simulink model "obserwator_stanu"  (R2022b)
settings: Solver=ode3  StartTime=0.0  StopTime=1  FixedStep=Tp  RelTol=1e-3
values from neighbouring files (symbols this model uses):
  A = [0 1 0; a21 0 a23; a31 0 a33]    [init.m]    (also in proj.m)
  a21 = 1/2/m * x30^2 * FemP1/FemP2^2 * exp(-x10/FemP2)    [init.m]    (also in proj.m)
  a23 = -1/m * x30 * FemP1/FemP2 * exp(-x10/FemP2)    [init.m]    (also in proj.m)
  a31 = 1/f1 * exp(x10/f2) * (ki*u10 + ci - x30)    [init.m]    (also in proj.m)
  a33 = -f2/f1 * exp(x10/f2)    [init.m]    (also in proj.m)
  B = [0 0; 0 g; b31 0]    [init.m]    (also in proj.m)
  b31 = ki * f2/f1 * exp(x10/f2)    [init.m]    (also in proj.m)
  C = [1 0 0]    [init.m]    (also in proj.m)
  g = 9.81    [init.m]    (also in proj.m)
  K = place(A, B(:, 1), [-28, -60, -90])    [init.m]    (also in proj.m)
  L = acker(A', C', p)'    [init.m]    (also in proj.m)
  Tp = 0.00001    (= 1e-05)    [init.m]    (also in proj.m)
  xd = d-bd    [init.m]    (also in proj.m)
settings Model: Creator=TheZl  LastModifiedBy=minekuba

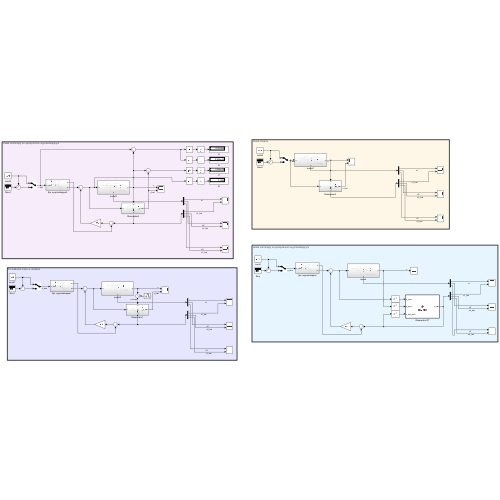
[thumbnail: Simulink's stored preview of the top-level diagram]
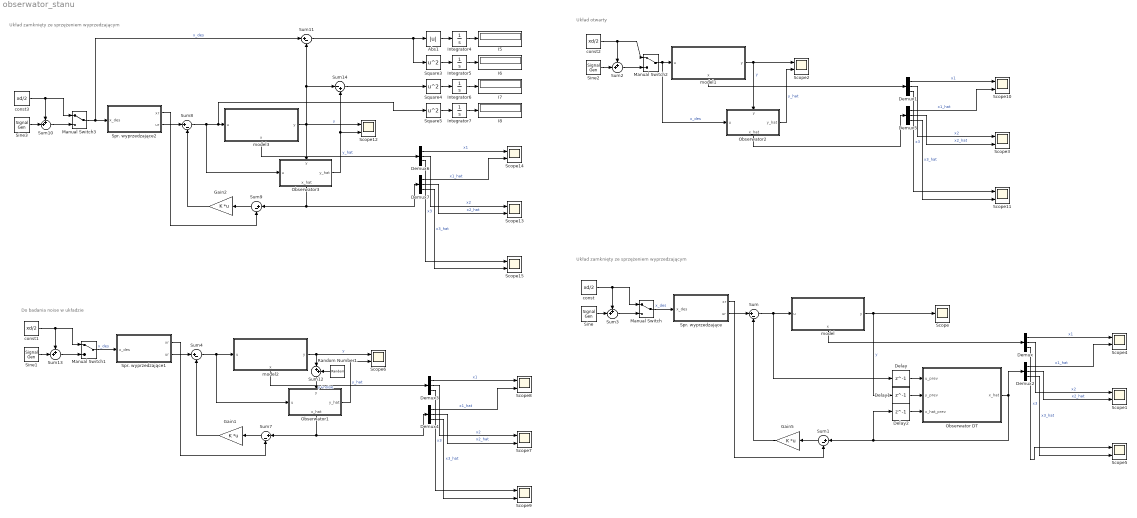
== system obserwator_stanu ==
  note: Układ zamknięty ze sprzężeniem wyprzedzającym
  note: Do badania noise w układzie
  note: Układ otwarty
  note: Układ zamknięty ze sprzężeniem wyprzedzającym
  Abs1 : Abs  SaturateOnIntegerOverflow=off
  Delay : Delay  DelayLength=1
  Delay1 : Delay  DelayLength=1
  Delay2 : Delay  DelayLength=1  InitialCondition=[0 0 0]'
  Demux{,1..7} (8 alike) : Demux  Outputs=3
  Gain1 : Gain  Gain=K  Multiplication=Matrix(K*u)
  Gain2 : Gain  Gain=K  Multiplication=Matrix(K*u)
  Gain5 : Gain  Gain=K  Multiplication=Matrix(K*u)
  I{5..8} (4 alike) : Display
  Integrator{4..7} (4 alike) : Integrator
  Manual Switch{,1..3} (4 alike) : ManualSwitch
  Obserwator DT : MATLAB Function  TreatAsAtomicUnit=on
  Obserwator1 : Subsystem
      settings: PortSchema="{\"entries\":[{\"content\":{\"sides\":[{\"content\":{\"connectorIds\":[\"In1\"]},\"type\":\"ConnectorPlacement.EquallySpacedRectSide\",\"uuid\":\"f0864749-42ee-43af-89d8-e79f181d54f0\"},{\"content\":{\"connectorIds\":[\"Out1\"],\"side\":\"RIGHT\"},\"type\":\"ConnectorPlacement.EquallySpacedRectSide\",\"uuid\":\"0332ef02-e2af-4e04-af5b-f19b3f506f90\"},{\"content\":{\"connectorIds\":[\"In2\"],\"side\":\"TOP\"},\"type\":\"ConnectorPlacement.EquallySpacedRectSide\",\"uuid\":\"17939e36-b316-45a4-8ef0-4ca25066d29d\"},{\"content\":{\"connectorIds\":[\"Out2\"],\"side\":\"BOTTOM\"},\"type\":\"ConnectorPlacement.EquallySpacedRectSide\",\"uuid\":\"291cc938-6a40-4d14-9d0d-6f037a5c762b\"}]},\"type\":\"ConnectorPlacement.EquallySpacedConnector\",\"uuid\":\"9ac518b4-bfcb-4f10-b20b-cf60c9eac4c7\"}],\"packageUris\":[\"http://schema.mathworks.com/mf0/Connector/R2020b\"],\"version\":\"1.0\"}"
  Obserwator2 : Subsystem
      settings: PortSchema="{\"entries\":[{\"content\":{\"sides\":[{\"content\":{\"connectorIds\":[\"In1\"]},\"type\":\"ConnectorPlacement.EquallySpacedRectSide\",\"uuid\":\"f0864749-42ee-43af-89d8-e79f181d54f0\"},{\"content\":{\"connectorIds\":[\"Out1\"],\"side\":\"RIGHT\"},\"type\":\"ConnectorPlacement.EquallySpacedRectSide\",\"uuid\":\"0332ef02-e2af-4e04-af5b-f19b3f506f90\"},{\"content\":{\"connectorIds\":[\"In2\"],\"side\":\"TOP\"},\"type\":\"ConnectorPlacement.EquallySpacedRectSide\",\"uuid\":\"17939e36-b316-45a4-8ef0-4ca25066d29d\"},{\"content\":{\"connectorIds\":[\"Out2\"],\"side\":\"BOTTOM\"},\"type\":\"ConnectorPlacement.EquallySpacedRectSide\",\"uuid\":\"291cc938-6a40-4d14-9d0d-6f037a5c762b\"}]},\"type\":\"ConnectorPlacement.EquallySpacedConnector\",\"uuid\":\"9ac518b4-bfcb-4f10-b20b-cf60c9eac4c7\"}],\"packageUris\":[\"http://schema.mathworks.com/mf0/Connector/R2020b\"],\"version\":\"1.0\"}"
  Obserwator3 : Subsystem
      settings: PortSchema="{\"entries\":[{\"content\":{\"sides\":[{\"content\":{\"connectorIds\":[\"In1\"]},\"type\":\"ConnectorPlacement.EquallySpacedRectSide\",\"uuid\":\"f0864749-42ee-43af-89d8-e79f181d54f0\"},{\"content\":{\"connectorIds\":[\"Out1\"],\"side\":\"RIGHT\"},\"type\":\"ConnectorPlacement.EquallySpacedRectSide\",\"uuid\":\"0332ef02-e2af-4e04-af5b-f19b3f506f90\"},{\"content\":{\"connectorIds\":[\"In2\"],\"side\":\"TOP\"},\"type\":\"ConnectorPlacement.EquallySpacedRectSide\",\"uuid\":\"17939e36-b316-45a4-8ef0-4ca25066d29d\"},{\"content\":{\"connectorIds\":[\"Out2\"],\"side\":\"BOTTOM\"},\"type\":\"ConnectorPlacement.EquallySpacedRectSide\",\"uuid\":\"291cc938-6a40-4d14-9d0d-6f037a5c762b\"}]},\"type\":\"ConnectorPlacement.EquallySpacedConnector\",\"uuid\":\"9ac518b4-bfcb-4f10-b20b-cf60c9eac4c7\"}],\"packageUris\":[\"http://schema.mathworks.com/mf0/Connector/R2020b\"],\"version\":\"1.0\"}"
  Random Number1 : RandomNumber  Variance=1e-5
  Scope : Scope
  Scope{1..15} (15 alike) : Scope  NumInputPorts=2
  Sine{,1..3} (4 alike) : SignalGenerator  Amplitude=xd/12  Frequency=0.2
  Spr. wyprzedzające : Subsystem
  Spr. wyprzedzające1 : Subsystem
  Spr. wyprzedzające2 : Subsystem
  Square3 : Math  Operator=square
  Square4 : Math  Operator=square
  Square5 : Math  Operator=square
  Sum{,1,4,7..9,11} (7 alike) : Sum  Inputs=|+-
  Sum{2..3,10,13} (4 alike) : Sum  Inputs=++|
  Sum12 : Sum  Inputs=|++
  Sum14 : Sum  Inputs=|-+
  const{,1..3} (4 alike) : Constant  Value=xd/2
  model : Subsystem
      settings: PortSchema="{\"entries\":[{\"content\":{\"sides\":[{\"content\":{\"connectorIds\":[\"In1\"]},\"type\":\"ConnectorPlacement.EquallySpacedRectSide\",\"uuid\":\"08100310-f669-4bec-b75a-4c341ab1329c\"},{\"content\":{\"connectorIds\":[\"Out1\"],\"side\":\"RIGHT\"},\"type\":\"ConnectorPlacement.EquallySpacedRectSide\",\"uuid\":\"75a75395-bc88-4968-acfb-02365cdbbaac\"},{\"content\":{\"connectorIds\":[],\"side\":\"TOP\"},\"type\":\"ConnectorPlacement.EquallySpacedRectSide\",\"uuid\":\"7e90434d-1931-47ff-b270-f1d54f71bb7e\"},{\"content\":{\"connectorIds\":[\"Out2\"],\"side\":\"BOTTOM\"},\"type\":\"ConnectorPlacement.EquallySpacedRectSide\",\"uuid\":\"09ce4af7-043c-4542-961c-50c1fb378fc1\"}]},\"type\":\"ConnectorPlacement.EquallySpacedConnector\",\"uuid\":\"9c93e3e1-5fb5-4a02-9a28-f46059e1f065\"}],\"packageUris\":[\"http://schema.mathworks.com/mf0/Connector/R2020b\"],\"version\":\"1.0\"}"
  model1 : Subsystem
      settings: PortSchema="{\"entries\":[{\"content\":{\"sides\":[{\"content\":{\"connectorIds\":[\"In1\"]},\"type\":\"ConnectorPlacement.EquallySpacedRectSide\",\"uuid\":\"08100310-f669-4bec-b75a-4c341ab1329c\"},{\"content\":{\"connectorIds\":[\"Out1\"],\"side\":\"RIGHT\"},\"type\":\"ConnectorPlacement.EquallySpacedRectSide\",\"uuid\":\"75a75395-bc88-4968-acfb-02365cdbbaac\"},{\"content\":{\"connectorIds\":[],\"side\":\"TOP\"},\"type\":\"ConnectorPlacement.EquallySpacedRectSide\",\"uuid\":\"7e90434d-1931-47ff-b270-f1d54f71bb7e\"},{\"content\":{\"connectorIds\":[\"Out2\"],\"side\":\"BOTTOM\"},\"type\":\"ConnectorPlacement.EquallySpacedRectSide\",\"uuid\":\"09ce4af7-043c-4542-961c-50c1fb378fc1\"}]},\"type\":\"ConnectorPlacement.EquallySpacedConnector\",\"uuid\":\"9c93e3e1-5fb5-4a02-9a28-f46059e1f065\"}],\"packageUris\":[\"http://schema.mathworks.com/mf0/Connector/R2020b\"],\"version\":\"1.0\"}"
  model2 : Subsystem
      settings: PortSchema="{\"entries\":[{\"content\":{\"sides\":[{\"content\":{\"connectorIds\":[\"In1\"]},\"type\":\"ConnectorPlacement.EquallySpacedRectSide\",\"uuid\":\"08100310-f669-4bec-b75a-4c341ab1329c\"},{\"content\":{\"connectorIds\":[\"Out1\"],\"side\":\"RIGHT\"},\"type\":\"ConnectorPlacement.EquallySpacedRectSide\",\"uuid\":\"75a75395-bc88-4968-acfb-02365cdbbaac\"},{\"content\":{\"connectorIds\":[],\"side\":\"TOP\"},\"type\":\"ConnectorPlacement.EquallySpacedRectSide\",\"uuid\":\"7e90434d-1931-47ff-b270-f1d54f71bb7e\"},{\"content\":{\"connectorIds\":[\"Out2\"],\"side\":\"BOTTOM\"},\"type\":\"ConnectorPlacement.EquallySpacedRectSide\",\"uuid\":\"09ce4af7-043c-4542-961c-50c1fb378fc1\"}]},\"type\":\"ConnectorPlacement.EquallySpacedConnector\",\"uuid\":\"9c93e3e1-5fb5-4a02-9a28-f46059e1f065\"}],\"packageUris\":[\"http://schema.mathworks.com/mf0/Connector/R2020b\"],\"version\":\"1.0\"}"
  model3 : Subsystem
      settings: PortSchema="{\"entries\":[{\"content\":{\"sides\":[{\"content\":{\"connectorIds\":[\"In1\"]},\"type\":\"ConnectorPlacement.EquallySpacedRectSide\",\"uuid\":\"08100310-f669-4bec-b75a-4c341ab1329c\"},{\"content\":{\"connectorIds\":[\"Out1\"],\"side\":\"RIGHT\"},\"type\":\"ConnectorPlacement.EquallySpacedRectSide\",\"uuid\":\"75a75395-bc88-4968-acfb-02365cdbbaac\"},{\"content\":{\"connectorIds\":[],\"side\":\"TOP\"},\"type\":\"ConnectorPlacement.EquallySpacedRectSide\",\"uuid\":\"7e90434d-1931-47ff-b270-f1d54f71bb7e\"},{\"content\":{\"connectorIds\":[\"Out2\"],\"side\":\"BOTTOM\"},\"type\":\"ConnectorPlacement.EquallySpacedRectSide\",\"uuid\":\"09ce4af7-043c-4542-961c-50c1fb378fc1\"}]},\"type\":\"ConnectorPlacement.EquallySpacedConnector\",\"uuid\":\"9c93e3e1-5fb5-4a02-9a28-f46059e1f065\"}],\"packageUris\":[\"http://schema.mathworks.com/mf0/Connector/R2020b\"],\"version\":\"1.0\"}"
  wires:
  model/1(y) -> Delay1/1, Scope/1  "y"
  Sum/1 -> model/1(u), Delay/1
  Gain5/1 -> Sum/2
  Sum3/1 -> Manual Switch/2
  const/1 -> Sum3/1, Manual Switch/1
  Sine/1 -> Sum3/2
  Manual Switch/1 -> Spr. wyprzedzające/1(x_des)  "x_des"
  Spr. wyprzedzające/2(ur) -> Sum/1
  Spr. wyprzedzające/1(xr) -> Sum1/2
  model/2(x) -> Demux/1
  Demux/1 -> Scope4/1  "x1"
  Demux2/1 -> Scope4/2  "x1_hat"
  Demux/2 -> Scope1/1  "x2"
  Demux2/2 -> Scope1/2  "x2_hat"
  Demux/3 -> Scope5/1  "x3"
  Demux2/3 -> Scope5/2  "x3_hat"
  const1/1 -> Sum13/1, Manual Switch1/1
  Sum13/1 -> Manual Switch1/2
  Gain1/1 -> Sum4/2
  Spr. wyprzedzające1/2(ur) -> Sum4/1
  Demux3/1 -> Scope8/1  "x1"
  Demux4/2 -> Scope7/2  "x2_hat"
  model2/1(y) -> Sum12/1, Scope6/1  "y"
  Manual Switch1/1 -> Spr. wyprzedzające1/1(x_des)  "x_des"
  Sine1/1 -> Sum13/2
  Demux4/1 -> Scope8/2  "x1_hat"
  Obserwator1/2(x_hat) -> Demux4/1, Sum7/1
  Obserwator1/1(y_hat) -> Scope6/2  "y_hat"
  Spr. wyprzedzające1/1(xr) -> Sum7/2
  Sum4/1 -> Obserwator1/1(u), model2/1(u)
  model2/2(x) -> Demux3/1
  Demux3/3 -> Scope9/1  "x3"
  Sum7/1 -> Gain1/1
  Demux4/3 -> Scope9/2  "x3_hat"
  Demux3/2 -> Scope7/1  "x2"
  Sum12/1 -> Obserwator1/2(y)  "y+noise"
  Random Number1/1 -> Sum12/2
  model1/1(y) -> Scope2/1, Obserwator2/2(y)  "y"
  Manual Switch2/1 -> Obserwator2/1(u), model1/1(u)  "x_des"
  const2/1 -> Sum2/1, Manual Switch2/1
  Sine2/1 -> Sum2/2
  Sum2/1 -> Manual Switch2/2
  Demux5/2 -> Scope3/2  "x2_hat"
  Demux1/1 -> Scope10/1  "x1"
  Demux5/1 -> Scope10/2  "x1_hat"
  Demux1/3 -> Scope11/1  "x3"
  Demux5/3 -> Scope11/2  "x3_hat"
  Demux1/2 -> Scope3/1  "x2"
  model1/2(x) -> Demux1/1
  Obserwator2/2(x_hat) -> Demux5/1
  Obserwator2/1(y_hat) -> Scope2/2  "y_hat"
  Square4/1 -> Integrator6/1
  Integrator6/1 -> I7/1
  Square3/1 -> Integrator5/1
  Integrator7/1 -> I8/1
  Integrator5/1 -> I6/1
  Abs1/1 -> Integrator4/1
  const3/1 -> Sum10/1, Manual Switch3/1
  Sum10/1 -> Manual Switch3/2
  Gain2/1 -> Sum8/2
  Spr. wyprzedzające2/2(ur) -> Sum8/1
  Demux6/1 -> Scope14/1  "x1"
  Demux7/2 -> Scope13/2  "x2_hat"
  Sum11/1 -> Abs1/1, Square3/1
  Square5/1 -> Integrator7/1
  Sine3/1 -> Sum10/2
  Manual Switch3/1 -> Sum11/1, Spr. wyprzedzające2/1(x_des)  "x_des"
  Demux7/1 -> Scope14/2  "x1_hat"
  Sum14/1 -> Square4/1
  model3/1(y) -> Scope12/1, Sum11/2, Sum14/1, Obserwator3/2(y)  "y"
  Obserwator3/2(x_hat) -> Demux7/1, Sum9/1
  Integrator4/1 -> I5/1
  Obserwator3/1(y_hat) -> Sum14/2, Scope12/2  "y_hat"
  Spr. wyprzedzające2/1(xr) -> Sum9/2
  Sum8/1 -> Square5/1, model3/1(u), Obserwator3/1(u)
  model3/2(x) -> Demux6/1
  Demux6/3 -> Scope15/1  "x3"
  Sum9/1 -> Gain2/1
  Demux7/3 -> Scope15/2  "x3_hat"
  Demux6/2 -> Scope13/1  "x2"
  Obserwator DT/1(x_hat) -> Demux2/1, Delay2/1, Sum1/1
  Sum1/1 -> Gain5/1
  Delay/1 -> Obserwator DT/1(u_prev)
  Delay1/1 -> Obserwator DT/2(y_prev)
  Delay2/1 -> Obserwator DT/3(x_hat_prev)

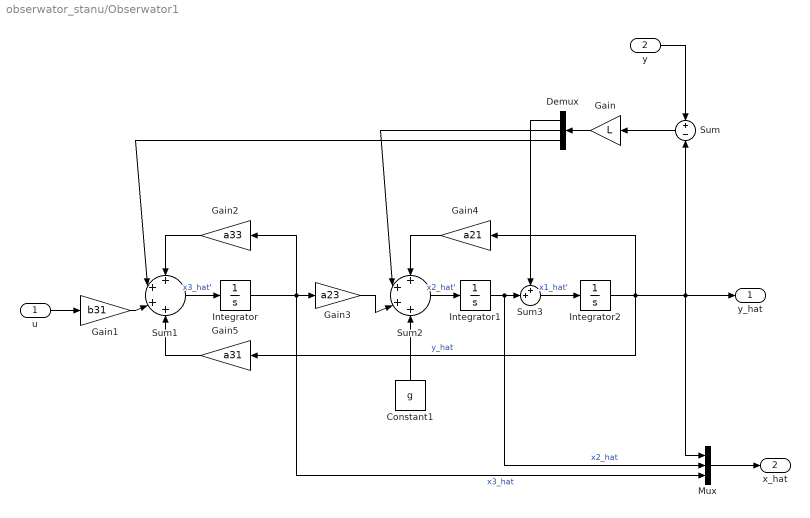
== system obserwator_stanu/Obserwator1 ==
  u : Inport
  y : Inport  Port=2
  Constant1 : Constant  Value=g
  Demux : Demux  Outputs=3
  Gain : Gain  Gain=L
  Gain1 : Gain  Gain=b31
  Gain2 : Gain  Gain=a33
  Gain3 : Gain  Gain=a23
  Gain4 : Gain  Gain=a21
  Gain5 : Gain  Gain=a31
  Integrator : Integrator
  Integrator1 : Integrator
  Integrator2 : Integrator  UpperSaturationLimit=xd  LowerSaturationLimit=0
  Mux : Mux  Inputs=3
  Sum : Sum  Inputs=+|-
  Sum1 : Sum  Inputs=++++
  Sum2 : Sum  Inputs=++++
  Sum3 : Sum  Inputs=++|
  y_hat : Outport
  x_hat : Outport  Port=2
  wires:
  Demux/1 -> Sum3/1
  Gain4/1 -> Sum2/1
  Sum2/1 -> Integrator1/1  "x2_hat'"
  Sum/1 -> Gain/1
  Gain3/1 -> Sum2/3
  Integrator2/1 -> Gain4/1, Mux/1, y_hat/1, Sum/2, Gain5/1  "y_hat"
  Gain1/1 -> Sum1/3
  Sum1/1 -> Integrator/1  "x3_hat'"
  Gain5/1 -> Sum1/4
  Gain/1 -> Demux/1
  Sum3/1 -> Integrator2/1  "x1_hat'"
  Gain2/1 -> Sum1/1
  Integrator1/1 -> Mux/2, Sum3/2  "x2_hat"
  Integrator/1 -> Mux/3, Gain2/1, Gain3/1  "x3_hat"
  Demux/2 -> Sum2/2
  Constant1/1 -> Sum2/4
  Demux/3 -> Sum1/2
  y/1 -> Sum/1
  u/1 -> Gain1/1
  Mux/1 -> x_hat/1

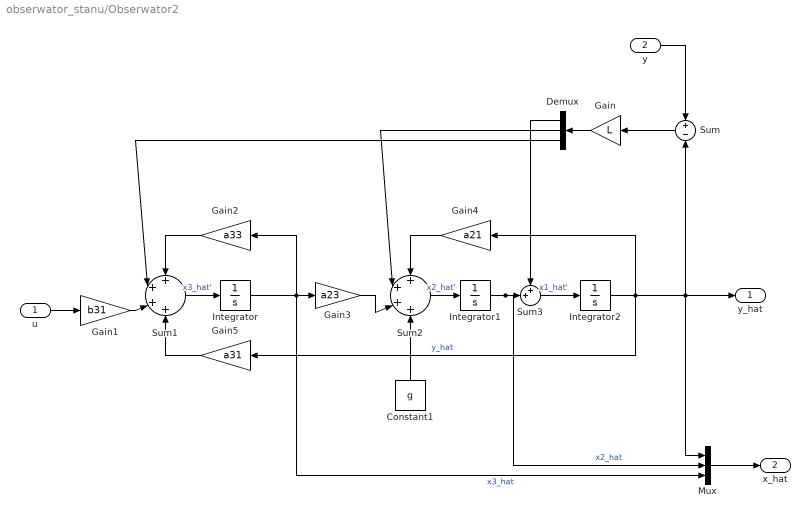
== system obserwator_stanu/Obserwator2 ==
  u : Inport
  y : Inport  Port=2
  Constant1 : Constant  Value=g
  Demux : Demux  Outputs=3
  Gain : Gain  Gain=L
  Gain1 : Gain  Gain=b31
  Gain2 : Gain  Gain=a33
  Gain3 : Gain  Gain=a23
  Gain4 : Gain  Gain=a21
  Gain5 : Gain  Gain=a31
  Integrator : Integrator
  Integrator1 : Integrator
  Integrator2 : Integrator  UpperSaturationLimit=xd  LowerSaturationLimit=0
  Mux : Mux  Inputs=3
  Sum : Sum  Inputs=+|-
  Sum1 : Sum  Inputs=++++
  Sum2 : Sum  Inputs=++++
  Sum3 : Sum  Inputs=++|
  y_hat : Outport
  x_hat : Outport  Port=2
  wires:
  Demux/1 -> Sum3/1
  Gain4/1 -> Sum2/1
  Sum2/1 -> Integrator1/1  "x2_hat'"
  Sum/1 -> Gain/1
  Gain3/1 -> Sum2/3
  Integrator2/1 -> Gain4/1, Mux/1, y_hat/1, Sum/2, Gain5/1  "y_hat"
  Gain1/1 -> Sum1/3
  Sum1/1 -> Integrator/1  "x3_hat'"
  Gain5/1 -> Sum1/4
  Gain/1 -> Demux/1
  Sum3/1 -> Integrator2/1  "x1_hat'"
  Gain2/1 -> Sum1/1
  Integrator1/1 -> Mux/2, Sum3/2  "x2_hat"
  Integrator/1 -> Mux/3, Gain2/1, Gain3/1  "x3_hat"
  Demux/2 -> Sum2/2
  Constant1/1 -> Sum2/4
  Demux/3 -> Sum1/2
  y/1 -> Sum/1
  u/1 -> Gain1/1
  Mux/1 -> x_hat/1

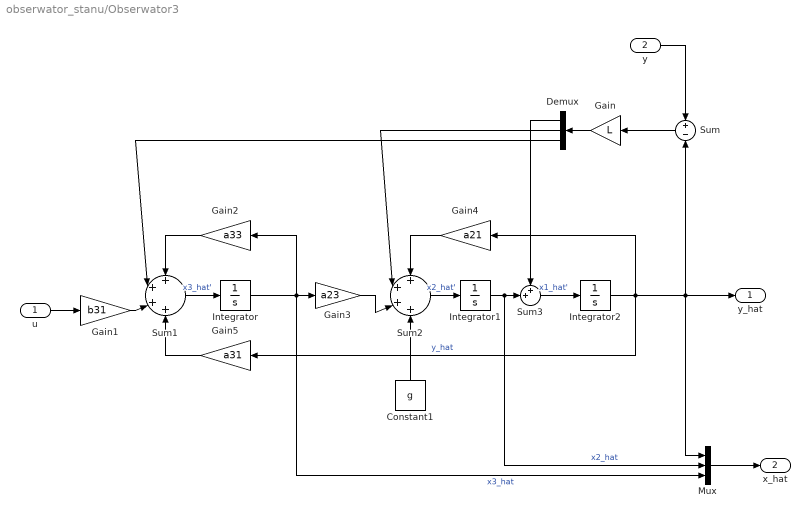
== system obserwator_stanu/Obserwator3 ==
  u : Inport
  y : Inport  Port=2
  Constant1 : Constant  Value=g
  Demux : Demux  Outputs=3
  Gain : Gain  Gain=L
  Gain1 : Gain  Gain=b31
  Gain2 : Gain  Gain=a33
  Gain3 : Gain  Gain=a23
  Gain4 : Gain  Gain=a21
  Gain5 : Gain  Gain=a31
  Integrator : Integrator
  Integrator1 : Integrator
  Integrator2 : Integrator  UpperSaturationLimit=xd  LowerSaturationLimit=0
  Mux : Mux  Inputs=3
  Sum : Sum  Inputs=+|-
  Sum1 : Sum  Inputs=++++
  Sum2 : Sum  Inputs=++++
  Sum3 : Sum  Inputs=++|
  y_hat : Outport
  x_hat : Outport  Port=2
  wires:
  Demux/1 -> Sum3/1
  Gain4/1 -> Sum2/1
  Sum2/1 -> Integrator1/1  "x2_hat'"
  Sum/1 -> Gain/1
  Gain3/1 -> Sum2/3
  Integrator2/1 -> Gain4/1, Mux/1, y_hat/1, Sum/2, Gain5/1  "y_hat"
  Gain1/1 -> Sum1/3
  Sum1/1 -> Integrator/1  "x3_hat'"
  Gain5/1 -> Sum1/4
  Gain/1 -> Demux/1
  Sum3/1 -> Integrator2/1  "x1_hat'"
  Gain2/1 -> Sum1/1
  Integrator1/1 -> Mux/2, Sum3/2  "x2_hat"
  Integrator/1 -> Mux/3, Gain2/1, Gain3/1  "x3_hat"
  Demux/2 -> Sum2/2
  Constant1/1 -> Sum2/4
  Demux/3 -> Sum1/2
  y/1 -> Sum/1
  u/1 -> Gain1/1
  Mux/1 -> x_hat/1

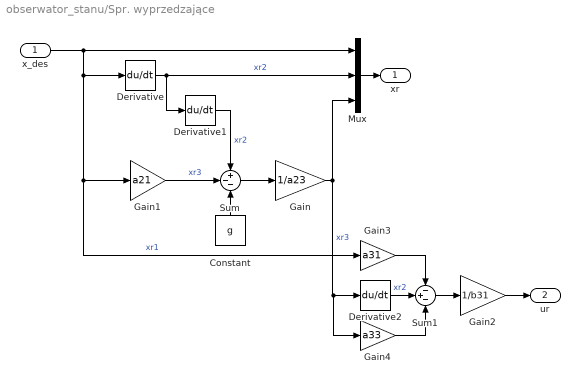
== system obserwator_stanu/Spr. wyprzedzające ==
  x_des : Inport
  Constant : Constant  Value=g
  Derivative : Derivative
  Derivative1 : Derivative
  Derivative2 : Derivative
  Gain : Gain  Gain=1/a23
  Gain1 : Gain  Gain=a21
  Gain2 : Gain  Gain=1/b31
  Gain3 : Gain  Gain=a31
  Gain4 : Gain  Gain=a33
  Mux : Mux  Inputs=3
  Sum : Sum  Inputs=+--
  Sum1 : Sum  Inputs=-+-
  xr : Outport
  ur : Outport  Port=2
  wires:
  Mux/1 -> xr/1
  x_des/1 -> Gain3/1, Gain1/1, Derivative/1, Mux/1  "xr1"
  Derivative/1 -> Derivative1/1, Mux/2  "xr2"
  Gain/1 -> Gain4/1, Derivative2/1, Mux/3  "xr3"
  Derivative1/1 -> Sum/1  "xr2"
  Sum/1 -> Gain/1
  Constant/1 -> Sum/3
  Gain1/1 -> Sum/2  "xr3"
  Gain2/1 -> ur/1
  Sum1/1 -> Gain2/1
  Derivative2/1 -> Sum1/2  "xr2"
  Gain3/1 -> Sum1/1
  Gain4/1 -> Sum1/3

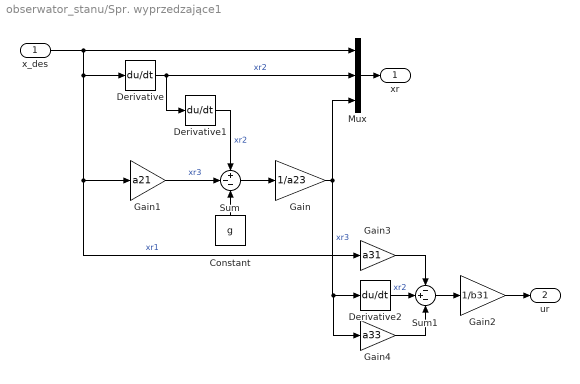
== system obserwator_stanu/Spr. wyprzedzające1 ==
  x_des : Inport
  Constant : Constant  Value=g
  Derivative : Derivative
  Derivative1 : Derivative
  Derivative2 : Derivative
  Gain : Gain  Gain=1/a23
  Gain1 : Gain  Gain=a21
  Gain2 : Gain  Gain=1/b31
  Gain3 : Gain  Gain=a31
  Gain4 : Gain  Gain=a33
  Mux : Mux  Inputs=3
  Sum : Sum  Inputs=+--
  Sum1 : Sum  Inputs=-+-
  xr : Outport
  ur : Outport  Port=2
  wires:
  Mux/1 -> xr/1
  x_des/1 -> Gain3/1, Gain1/1, Derivative/1, Mux/1  "xr1"
  Derivative/1 -> Derivative1/1, Mux/2  "xr2"
  Gain/1 -> Gain4/1, Derivative2/1, Mux/3  "xr3"
  Derivative1/1 -> Sum/1  "xr2"
  Sum/1 -> Gain/1
  Constant/1 -> Sum/3
  Gain1/1 -> Sum/2  "xr3"
  Gain2/1 -> ur/1
  Sum1/1 -> Gain2/1
  Derivative2/1 -> Sum1/2  "xr2"
  Gain3/1 -> Sum1/1
  Gain4/1 -> Sum1/3

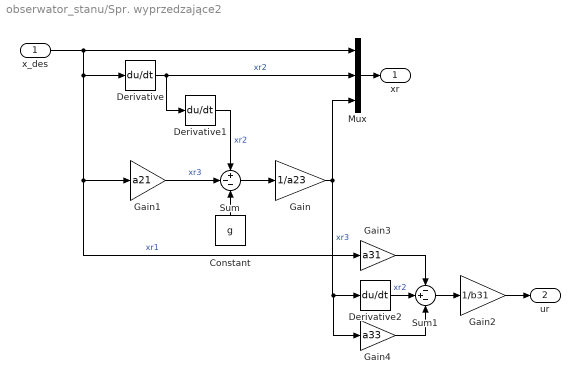
== system obserwator_stanu/Spr. wyprzedzające2 ==
  x_des : Inport
  Constant : Constant  Value=g
  Derivative : Derivative
  Derivative1 : Derivative
  Derivative2 : Derivative
  Gain : Gain  Gain=1/a23
  Gain1 : Gain  Gain=a21
  Gain2 : Gain  Gain=1/b31
  Gain3 : Gain  Gain=a31
  Gain4 : Gain  Gain=a33
  Mux : Mux  Inputs=3
  Sum : Sum  Inputs=+--
  Sum1 : Sum  Inputs=-+-
  xr : Outport
  ur : Outport  Port=2
  wires:
  Mux/1 -> xr/1
  x_des/1 -> Gain3/1, Gain1/1, Derivative/1, Mux/1  "xr1"
  Derivative/1 -> Derivative1/1, Mux/2  "xr2"
  Gain/1 -> Gain4/1, Derivative2/1, Mux/3  "xr3"
  Derivative1/1 -> Sum/1  "xr2"
  Sum/1 -> Gain/1
  Constant/1 -> Sum/3
  Gain1/1 -> Sum/2  "xr3"
  Gain2/1 -> ur/1
  Sum1/1 -> Gain2/1
  Derivative2/1 -> Sum1/2  "xr2"
  Gain3/1 -> Sum1/1
  Gain4/1 -> Sum1/3

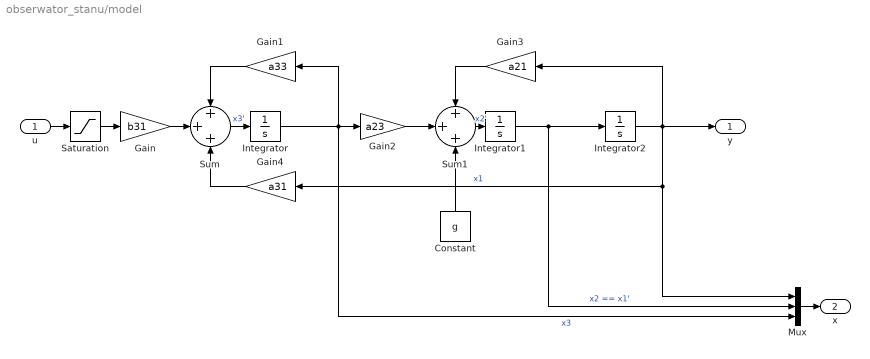
== system obserwator_stanu/model ==
  u : Inport
  Constant : Constant  Value=g
  Gain : Gain  Gain=b31
  Gain1 : Gain  Gain=a33
  Gain2 : Gain  Gain=a23
  Gain3 : Gain  Gain=a21
  Gain4 : Gain  Gain=a31
  Integrator : Integrator
  Integrator1 : Integrator
  Integrator2 : Integrator  InitialCondition=xd  LimitOutput=on  UpperSaturationLimit=xd  LowerSaturationLimit=0
  Mux : Mux  Inputs=3
  Saturation : Saturate  UpperLimit=1  LowerLimit=0
  Sum : Sum  Inputs=+++
  Sum1 : Sum  Inputs=+++
  y : Outport
  x : Outport  Port=2
  wires:
  Integrator2/1 -> y/1, Mux/1, Gain4/1, Gain3/1  "x1"
  Gain1/1 -> Sum/1
  Integrator/1 -> Mux/3, Gain2/1, Gain1/1  "x3"
  Constant/1 -> Sum1/3
  Gain/1 -> Sum/2
  Gain4/1 -> Sum/3
  u/1 -> Saturation/1
  Sum/1 -> Integrator/1  "x3'"
  Gain3/1 -> Sum1/1
  Sum1/1 -> Integrator1/1  "x2'"
  Saturation/1 -> Gain/1
  Gain2/1 -> Sum1/2
  Integrator1/1 -> Mux/2, Integrator2/1  "x2 == x1'"
  Mux/1 -> x/1

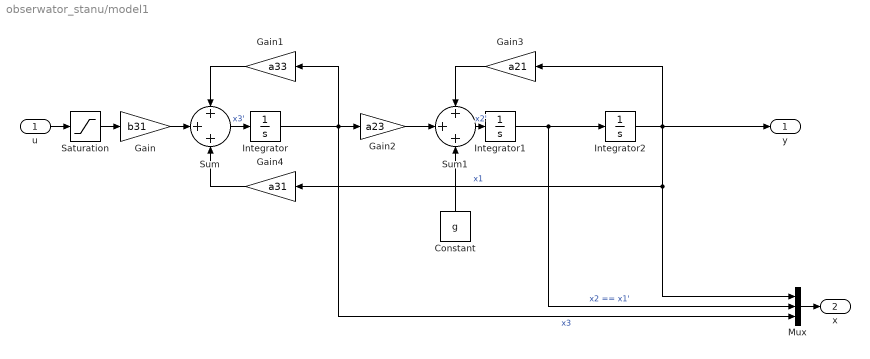
== system obserwator_stanu/model1 ==
  u : Inport
  Constant : Constant  Value=g
  Gain : Gain  Gain=b31
  Gain1 : Gain  Gain=a33
  Gain2 : Gain  Gain=a23
  Gain3 : Gain  Gain=a21
  Gain4 : Gain  Gain=a31
  Integrator : Integrator
  Integrator1 : Integrator
  Integrator2 : Integrator  InitialCondition=xd  LimitOutput=on  UpperSaturationLimit=xd  LowerSaturationLimit=0
  Mux : Mux  Inputs=3
  Saturation : Saturate  UpperLimit=1  LowerLimit=0
  Sum : Sum  Inputs=+++
  Sum1 : Sum  Inputs=+++
  y : Outport
  x : Outport  Port=2
  wires:
  Integrator2/1 -> y/1, Mux/1, Gain4/1, Gain3/1  "x1"
  Gain1/1 -> Sum/1
  Integrator/1 -> Mux/3, Gain2/1, Gain1/1  "x3"
  Constant/1 -> Sum1/3
  Gain/1 -> Sum/2
  Gain4/1 -> Sum/3
  u/1 -> Saturation/1
  Sum/1 -> Integrator/1  "x3'"
  Gain3/1 -> Sum1/1
  Sum1/1 -> Integrator1/1  "x2'"
  Saturation/1 -> Gain/1
  Gain2/1 -> Sum1/2
  Integrator1/1 -> Mux/2, Integrator2/1  "x2 == x1'"
  Mux/1 -> x/1

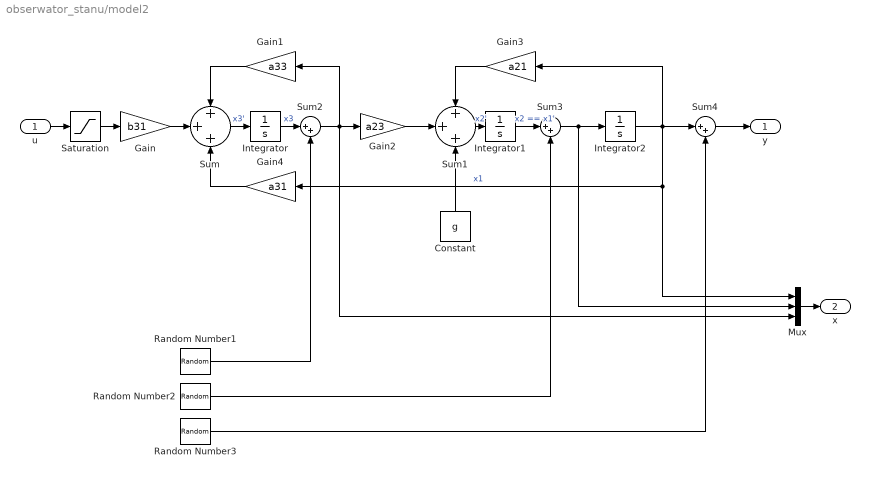
== system obserwator_stanu/model2 ==
  u : Inport
  Constant : Constant  Value=g
  Gain : Gain  Gain=b31
  Gain1 : Gain  Gain=a33
  Gain2 : Gain  Gain=a23
  Gain3 : Gain  Gain=a21
  Gain4 : Gain  Gain=a31
  Integrator : Integrator
  Integrator1 : Integrator
  Integrator2 : Integrator  InitialCondition=xd  LimitOutput=on  UpperSaturationLimit=xd  LowerSaturationLimit=0
  Mux : Mux  Inputs=3
  Random Number1 : RandomNumber  Variance=1e-3
  Random Number2 : RandomNumber  Variance=1e-4
  Random Number3 : RandomNumber  Variance=1e-5
  Saturation : Saturate  UpperLimit=1  LowerLimit=0
  Sum : Sum  Inputs=+++
  Sum1 : Sum  Inputs=+++
  Sum2 : Sum  Inputs=|++
  Sum3 : Sum  Inputs=|++
  Sum4 : Sum  Inputs=|++
  y : Outport
  x : Outport  Port=2
  wires:
  Integrator2/1 -> Sum4/1, Gain3/1, Mux/1, Gain4/1  "x1"
  Gain1/1 -> Sum/1
  Constant/1 -> Sum1/3
  Gain/1 -> Sum/2
  Gain4/1 -> Sum/3
  u/1 -> Saturation/1
  Sum/1 -> Integrator/1  "x3'"
  Gain3/1 -> Sum1/1
  Sum1/1 -> Integrator1/1  "x2'"
  Saturation/1 -> Gain/1
  Gain2/1 -> Sum1/2
  Mux/1 -> x/1
  Integrator/1 -> Sum2/1  "x3"
  Sum2/1 -> Mux/3, Gain1/1, Gain2/1
  Integrator1/1 -> Sum3/1  "x2 == x1'"
  Sum3/1 -> Mux/2, Integrator2/1
  Random Number2/1 -> Sum3/2
  Random Number1/1 -> Sum2/2
  Sum4/1 -> y/1
  Random Number3/1 -> Sum4/2

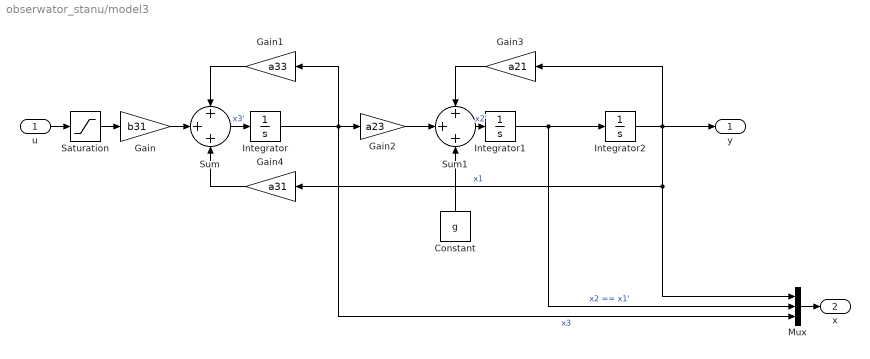
== system obserwator_stanu/model3 ==
  u : Inport
  Constant : Constant  Value=g
  Gain : Gain  Gain=b31
  Gain1 : Gain  Gain=a33
  Gain2 : Gain  Gain=a23
  Gain3 : Gain  Gain=a21
  Gain4 : Gain  Gain=a31
  Integrator : Integrator
  Integrator1 : Integrator
  Integrator2 : Integrator  InitialCondition=xd  LimitOutput=on  UpperSaturationLimit=xd  LowerSaturationLimit=0
  Mux : Mux  Inputs=3
  Saturation : Saturate  UpperLimit=1  LowerLimit=0
  Sum : Sum  Inputs=+++
  Sum1 : Sum  Inputs=+++
  y : Outport
  x : Outport  Port=2
  wires:
  Integrator2/1 -> y/1, Mux/1, Gain4/1, Gain3/1  "x1"
  Gain1/1 -> Sum/1
  Integrator/1 -> Mux/3, Gain2/1, Gain1/1  "x3"
  Constant/1 -> Sum1/3
  Gain/1 -> Sum/2
  Gain4/1 -> Sum/3
  u/1 -> Saturation/1
  Sum/1 -> Integrator/1  "x3'"
  Gain3/1 -> Sum1/1
  Sum1/1 -> Integrator1/1  "x2'"
  Saturation/1 -> Gain/1
  Gain2/1 -> Sum1/2
  Integrator1/1 -> Mux/2, Integrator2/1  "x2 == x1'"
  Mux/1 -> x/1

== matlab function obserwator_stanu/Obserwator DT ==
  data: x_hat output; u_prev input; y_prev input; x_hat_prev input; A parameter double; B parameter double; Tp parameter double; L parameter double; C parameter double
function x_hat = obsv_disc(u_prev, y_prev, x_hat_prev, A, B, Tp, L, C)
% assumes A, B, C, L, Tp are already defined
x_hat = (eye(length(A))+A*Tp)*x_hat_prev + B(:,1)*Tp*u_prev + L*Tp*(y_prev - C*x_hat_prev);
end
